simulink model "circuit2_starter"  (R2021b)
settings: Solver=VariableStepAuto  StartTime=0.0  StopTime=10.0  RelTol=1e-6
libraries: fl_lib x9, nesl_utility x1
settings Model: Creator=Rocksmithed  LastModifiedBy=Work

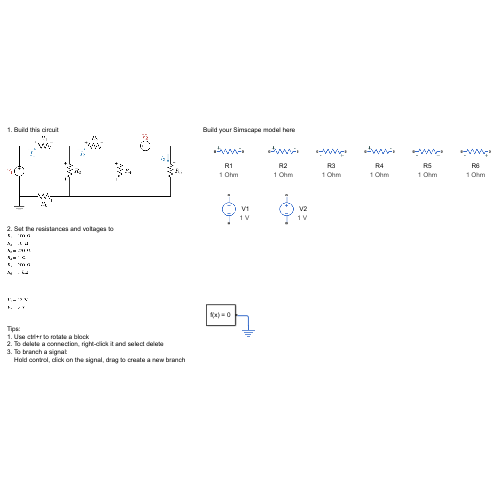
[thumbnail: Simulink's stored preview of the top-level diagram]
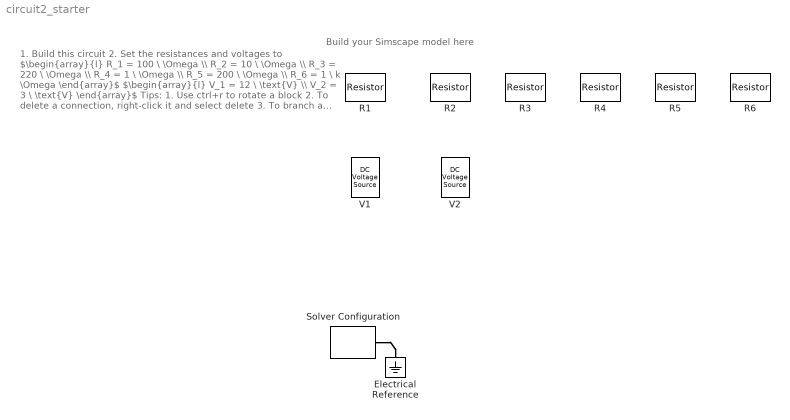
== system circuit2_starter ==
  note: 1. Build this circuit
      |
      | 2. Set the resistances and voltages to
      | $\begin{array}{l} R_1 = 100 \ \Omega \\ R_2 = 10 \ \Omega \\ R_3 = 220 \ \Omega \\ R_4 = 1 \ \Omega \\ R_5 = 200 \ \Omega \\ R_6 = 1 \ k \Omega \end{array}$
      | $\begin{array}{l} V_1 = 12 \ \text{V} \\ V_2 = 3 \ \text{V} \end{array}$
      |
      | Tips:
      | 1. Use ctrl+r to rotate a block
      | 2. To delete a connection, right-click it and select delete
      | 3. To branch a signal:
      | Hold control, click on the signal, drag to create a new branch
  note: Build your Simscape model here
  Electrical Reference : fl_lib/Electrical/Electrical Elements/Electrical Reference
  R{1..6} (6 alike) : fl_lib/Electrical/Electrical Elements/Resistor  R=1 Ohm  i_specify=off  i_priority=None  i=0 A  i_nominal_specify=off  i_nominal_unit=A  i_nominal_value=1  v_specify=off  v_priority=None  v=0 V  v_nominal_specify=off  v_nominal_unit=V  v_nominal_value=1
      settings: AttributesFormatString=%<R> %<R_unit>
  Solver Configuration : nesl_utility/Solver Configuration  PhysicalDomain=network_engine_domain  SubClassName=solver  LeftPortType=input  RightPortType=generic  Tones=[]  Harmonics=[]  SimulateNoise=off  Profile=off  UseLocalSampling=off  EnableSwitchedLinearOptims=on  FrequencyDomain=off  UseCCode=off  RelTol=0.001  AbsTol=1e-06  MinStep=1e-09  ToWorkspace=off  RevertToSquareIcSolve=off  NumHomotopyIterations=100  PhasorMode=off  PhasorModeNumHarmonics=1  DoDC=off  ResidualTolerance=1e-09  UseLocalSolver=off  LocalSolverChoice=NE_BACKWARD_EULER_ADVANCER  LocalSolverSampleTime=0.001  DoFixedCost=off  MaxNonlinIter=3  MaxModeIter=2  ComputeImpulses=off  ImpulseIterations=2  LinearAlgebra=auto  EquationFormulation=NE_TIME_EF  DelaysMemoryBudget=1024  AutomaticFiltering=on  FilteringTimeConstant=0.001  PartitionStorageMethod=AS_NEEDED  PartitionMemoryBudget=1024  PartitionMethod=ROBUST
      settings: SourceProductBaseCode=PW,SS
  V1 : fl_lib/Electrical/Electrical Sources/DC Voltage Source  v0=1 V
      settings: AttributesFormatString=%<v0> %<v0_unit>
  V2 : fl_lib/Electrical/Electrical Sources/DC Voltage Source  v0=1 V
      settings: AttributesFormatString=%<v0> %<v0_unit>
  connections:
  Solver Configuration/RConn1 -- Electrical Reference/LConn1
